simulink model "smriti_airgap_gamma"  (R2023a)
settings: Solver=VariableStepAuto  StartTime=0.0  StopTime=4  RelTol=1e-3
libraries: spsAsynchronousMachineSIUnitsLib x1, spsGroundLib x1, spsThreePhaseProgrammableVoltageSourceLib x1, spsThreePhaseVIMeasurementLib x1, spsThreePhaseBreakerLib x1, spsabctodq0Lib x1, sps_lib x1
settings Model: Creator=user  LastModifiedBy=user

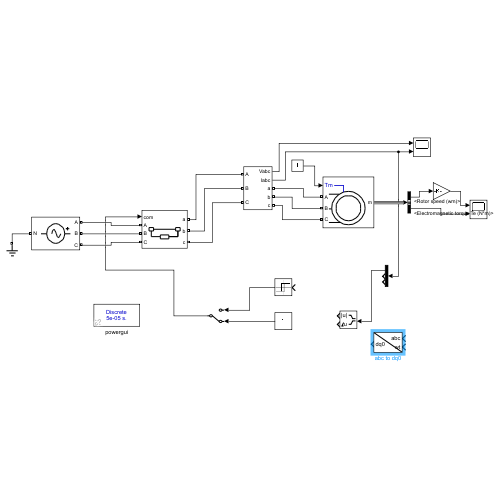
[thumbnail: Simulink's stored preview of the top-level diagram]
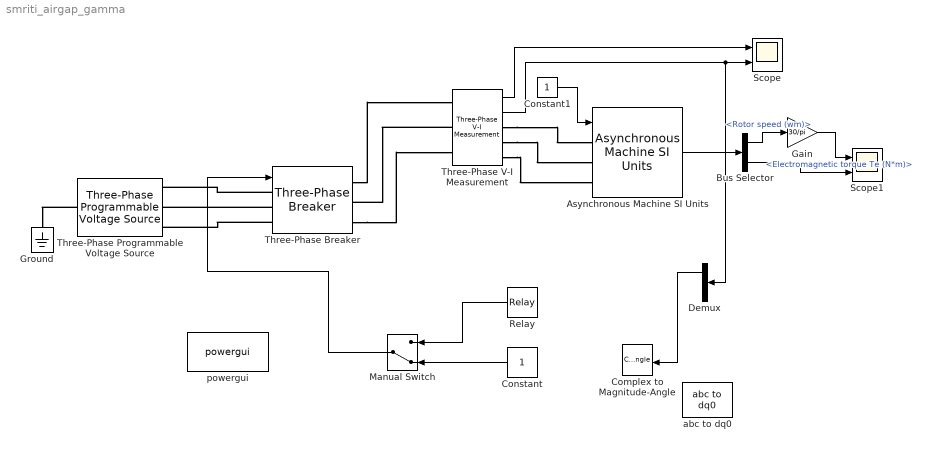
== system smriti_airgap_gamma ==
  Asynchronous Machine SI Units : spsAsynchronousMachineSIUnitsLib/Asynchronous Machine SI Units  RotorType=Squirrel-cage  PresetModel=No  MechanicalLoad=Torque Tm  ShowDetailedParameters=on  ReferenceFrame=Rotor  Units=SI  MeasurementBus=off  NominalParameters=[1.845e+04 400 50]  VoltageRatio=1  Stator=[0.5968 0.0003495]  Rotor=[0.6258 0.005473]  Cage1=[0.4155 0.002066]  Cage2=[0.4168 0.0003495]  Lm=0.0354  Mechanical=[0.05 0.005879 2]  PolePairs=2  InitialConditions=[0 0 0 0 0 0 0 0]  SimulateSaturation=off  Saturation=[14.03593122, 27.81365428, 53.79336849, 72.68890987, 97.98006896, 148.6815601, 215.7428561, 302.9841135, 428.7778367 ; 230, 322, 414, 460, 506, 552, 598, 644, 690]  LoadFlowParameters=1492000  TsPowergui=0  TsBlock=-1  IterativeModel=Trapezoidal non iterative  IterativeDiscreteModel=Trapezoidal non iterative  Pmec=1.492e+006
  Bus Selector : BusSelector  OutputSignals=Mechanical.Rotor speed (wm),Mechanical.Electromagnetic torque Te (N*m)
  Complex to Magnitude-Angle : ComplexToMagnitudeAngle
  Constant : Constant
  Constant1 : Constant
  Demux : Demux  Outputs=3
  Gain : Gain  Gain=30/pi
  Ground : spsGroundLib/Ground  LConnTagsString=a
  Manual Switch : ManualSwitch  CurrentSetting=0
  Relay : Relay
  Scope : Scope  NumInputPorts=2
  Scope1 : Scope  NumInputPorts=2
  Three-Phase Programmable Voltage Source : spsThreePhaseProgrammableVoltageSourceLib/Three-Phase Programmable Voltage Source  PositiveSequence="[400*sqrt(3)  0 60]"  VariationEntity=None  VariationType=Table of time-amplitude pairs  VariationTypeAlt=Step  VariationStep=0.5  VariationRate=10  VariationMagnitude=0.3  VariationFrequency=2  VariationTiming=[1 2]  VariationPhaseA=off  Amplitudes=[1 0.8 1.2 1.0]  TimeValues=[0 0.1 0.15 0.2]  HarmonicGeneration=off  HarmonicA=[3 0.2 -25 0]  HarmonicB=[2 0.15 35 2]  Timing="[0.05  3]"  BusType=swing  Pref=0  Qref=0  Qmin=-inf  Qmax=inf
  Three-Phase V-I Measurement : spsThreePhaseVIMeasurementLib/Three-Phase V-I Measurement  VoltageMeasurement=phase-to-phase  SetLabelV=off  LabelV=Vabc  Vpu=off  VpuLL=off  CurrentMeasurement=yes  SetLabelI=off  LabelI=Iabc  Ipu=off  Pbase=100e6  Vbase=500e3  OutputType=Complex  PhasorSimulation=off  PSBequivalent=0
  Three-Phase Breaker : spsThreePhaseBreakerLib/Three-Phase Breaker  InitialState=closed  SwitchA=on  SwitchB=on  SwitchC=on  SwitchTimes="[1/60  5/60]"  External=on  BreakerResistance=0.01  SnubberResistance=1e6  SnubberCapacitance=inf  Measurements=None
  abc to dq0 : spsabctodq0Lib/abc to dq0  Alignment=90 degrees behind phase A axis
  powergui : sps_lib/powergui  Priority=1  SimulationMode=Discrete  SampleTime=50e-6  frequency=60  Iterations=50  frequencyindice=50  Pbase=100e6  ErrMax=1e-4  UnitsV=kV  UnitsW=MW  buscounter=0  FunctionMessages=off  echomessages=off  EnableUseOfTLC=off  CurrentSourceSwitches=off  DisableSnubberDevices=off  DisableRonSwitches=off  DisableVfSwitches=off  DisplayEquations=off  AutomaticDiscreteSolvers=off  SolverType=Tustin/Backward Euler (TBE)  Interpol=off  ExternalGateDelay=off  methode=off  Ts=100  x0status=blocks  SPID=on  SwTol=0  HookPort=off  NonlinearTolerance=1e-4  nMaxIteration=100  ContinueOnMaxIteration=off  RestoreLinks=warning  ResistiveCurrentMeasurement=off  Frange=[0:2:500]  Ylog=off  Xlog=on  ShowGrid=off  save=off  variable=ZData  structure=0  ZoomFFT=off  StartTime=0.0  cycles=1  DisplayStyle=1  fundamental=60  FreqAxis=off  MaxFrequency=1000  frequencyindicesteady=1  RmsSteady=1  display=off
  wires:
  Constant/1 -> Manual Switch/2
  Relay/1 -> Manual Switch/1
  Constant1/1 -> Asynchronous Machine SI Units/1
  Three-Phase V-I Measurement/1 -> Scope/1
  Three-Phase V-I Measurement/2 -> Demux/1, Scope/2
  Manual Switch/1 -> Three-Phase Breaker/1
  Demux/1 -> Complex to Magnitude-Angle/1
  Asynchronous Machine SI Units/1 -> Bus Selector/1
  Bus Selector/1 -> Gain/1  "<Rotor speed (wm)>"
  Gain/1 -> Scope1/1
  Bus Selector/2 -> Scope1/2  "<Electromagnetic torque Te (N*m)>"
  connections:
  Three-Phase Breaker/RConn1 -- Three-Phase V-I Measurement/LConn1
  Three-Phase V-I Measurement/LConn2 -- Three-Phase Breaker/RConn2
  Three-Phase Breaker/RConn3 -- Three-Phase V-I Measurement/LConn3
  Three-Phase V-I Measurement/RConn1 -- Asynchronous Machine SI Units/LConn1
  Three-Phase V-I Measurement/RConn2 -- Asynchronous Machine SI Units/LConn2
  Three-Phase V-I Measurement/RConn3 -- Asynchronous Machine SI Units/LConn3
  Three-Phase Breaker/LConn1 -- Three-Phase Programmable Voltage Source/RConn1
  Three-Phase Breaker/LConn2 -- Three-Phase Programmable Voltage Source/RConn2
  Three-Phase Breaker/LConn3 -- Three-Phase Programmable Voltage Source/RConn3
  Three-Phase Programmable Voltage Source/LConn1 -- Ground/LConn1
